simulink model "antiwindup_main_PP"  (R2015a)
settings: Solver=ode45  StartTime=0.0  StopTime=10.0  RelTol=1e-3
undefined symbols (not defined in the file): sample
settings Model: Creator=teme  LastModifiedBy=teme

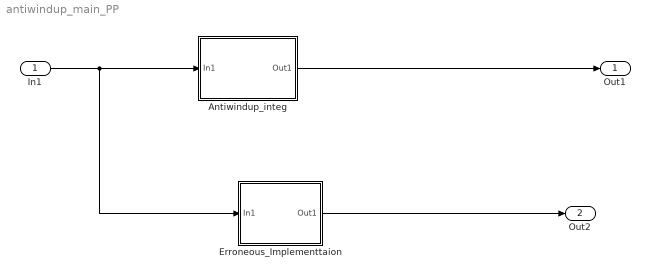
== system antiwindup_main_PP ==
  In1 : Inport  OutDataTypeStr=double
  Antiwindup_integ : Subsystem  TreatAsAtomicUnit=on
  Erroneous_Implementtaion : Subsystem  TreatAsAtomicUnit=on
  Out1 : Outport
  Out2 : Outport  Port=2
  wires:
  Antiwindup_integ/1(Out1) -> Out1/1
  In1/1 -> Erroneous_Implementtaion/1(In1), Antiwindup_integ/1(In1)
  Erroneous_Implementtaion/1(Out1) -> Out2/1

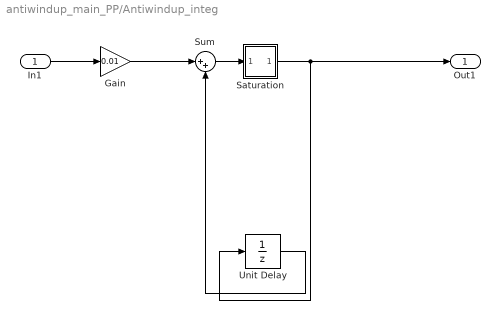
== system antiwindup_main_PP/Antiwindup_integ ==
  In1 : Inport  OutDataTypeStr=double
  Gain : Gain  Gain=0.01
  Saturation : Subsystem  TreatAsAtomicUnit=on
  Sum : Sum  Inputs=|++
  Unit Delay : UnitDelay  SampleTime=-1
  Out1 : Outport
  wires:
  Sum/1 -> Saturation/1(In)
  Gain/1 -> Sum/1
  Saturation/1(Out) -> Unit Delay/1, Out1/1
  Unit Delay/1 -> Sum/2
  In1/1 -> Gain/1

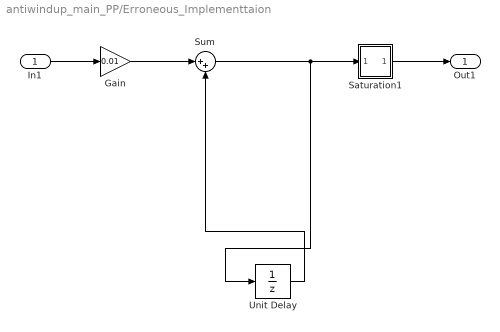
== system antiwindup_main_PP/Erroneous_Implementtaion ==
  In1 : Inport  OutDataTypeStr=double
  Gain : Gain  Gain=0.01
  Saturation1 : Subsystem  TreatAsAtomicUnit=on
  Sum : Sum  Inputs=|++
  Unit Delay : UnitDelay  SampleTime=-1
  Out1 : Outport
  wires:
  In1/1 -> Gain/1
  Unit Delay/1 -> Sum/2
  Gain/1 -> Sum/1
  Sum/1 -> Unit Delay/1, Saturation1/1(In)
  Saturation1/1(Out) -> Out1/1

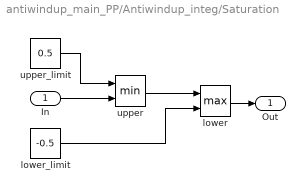
== system antiwindup_main_PP/Antiwindup_integ/Saturation ==
  In : Inport  OutDataTypeStr=double
  lower : MinMax  Function=max  Inputs=2
  lower_limit : Constant  Value=-0.5  SampleTime=0.1
  upper : MinMax  Inputs=2
  upper_limit : Constant  Value=0.5  SampleTime=0.1
  Out : Outport
  wires:
  lower/1 -> Out/1
  In/1 -> upper/2
  lower_limit/1 -> lower/2
  upper/1 -> lower/1
  upper_limit/1 -> upper/1

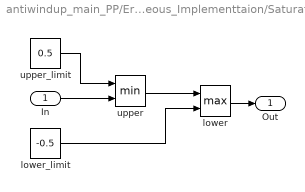
== system antiwindup_main_PP/Erroneous_Implementtaion/Saturation1 ==
  In : Inport  OutDataTypeStr=double
  lower : MinMax  Function=max  Inputs=2
  lower_limit : Constant  Value=-0.5  SampleTime=0.1
  upper : MinMax  Inputs=2
  upper_limit : Constant  Value=0.5  SampleTime=sample
  Out : Outport
  wires:
  lower/1 -> Out/1
  In/1 -> upper/2
  lower_limit/1 -> lower/2
  upper/1 -> lower/1
  upper_limit/1 -> upper/1
